simulink library "pfb_library"  (Simulink 6.2)
undefined symbols (not defined in the file or in its folder): add_latency, BitWidthIn, BitWidthOut, bram_latency, buf, CoeffBitWidth, n_inputs, PFBSize, TotalTaps, WindowType
libraries: xbsIndex_r3 x169, pfb_library x11
(part 1 of 2)
settings Model: LastModifiedBy=hchen05

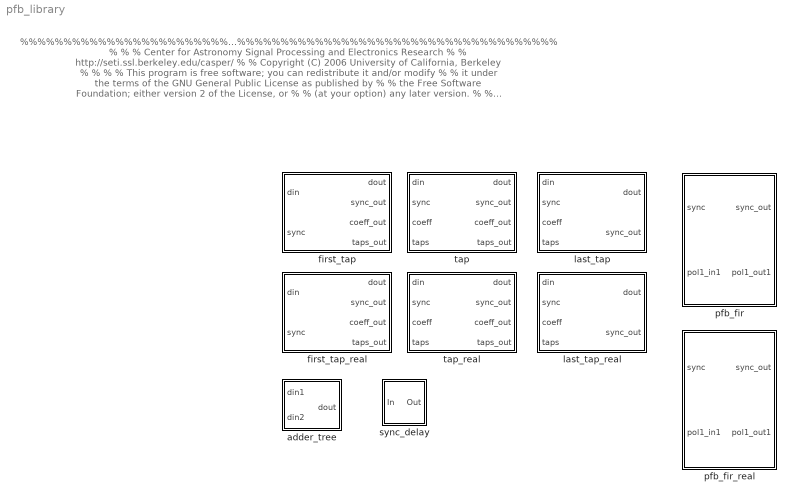
== system pfb_library ==
  note: %%%%%%%%%%%%%%%%%%%%%%%%%%%%%%%%%%%%%%%%%%%%%%%%%%%%%%%%%%%%%%%%%%%%%%%%%%%%%%%
      | %                                                                             %
      | %   Center for Astronomy Signal Processing and Electronics Research           %
      | %   http://seti.ssl.berkeley.edu/casper/                                      %
      | %   Copyright (C) 2006 University of California, Berkeley                     %
      | %                                                                             %
      | %   This program is free software; you can redistribute it and/or modify      %
      | %   it under the terms of the GNU General Public License as published by      %
      | %   the Free Software Foundation; either version 2 of the License, or         %
      | %   (at your option) any later version.                                       %
      | %                                                                             %
      | %   This program is distributed in the hope that it will be useful,           %
      | %   but WITHOUT ANY WARRANTY; without even the implied warranty of            %
      | %   MERCHANTABILITY or FITNESS FOR A PARTICULAR PURPOSE.  See the             %
      | %   GNU General Public License for more details.                              %
      | %                                                                             %
      | %   You should have received a copy of the GNU General Public License along   %
      | %   with this program; if not, write to the Free Software Foundation, Inc.,   %
      | %   51 Franklin Street, Fifth Floor, Boston, MA 02110-1301 USA.               %
      | %                                                                             %
      | %%%%%%%%%%%%%%%%%%%%%%%%%%%%%%%%%%%%%%%%%%%%%%%%%%%%%%%%%%%%%%%%%%%%%%%%%%%%%%%
  adder_tree : Subsystem  mask{num_inputs=2, latency=2}
      mask prompts: num_inputs "Inputs"; latency "Latency per adder tree"
      mask init:
      | adder_tree_mask;
  first_tap : Subsystem  mask(pfb_tap){nput=1, CoeffDistMem=off, fwidth=1}
      mask prompts: nput "This is input number:"; CoeffDistMem "Implement Coefficients in Distributed Memory"; fwidth "Bin Width (normal = 1)"
      mask init:
      | cursys = gcb;
      | disp(cursys);
      | if ~strcmp(get_param([cursys,'/pfb_coeff_gen'], 'CoeffDistMem'), CoeffDistMem),
      |     set_param([cursys,'/pfb_coeff_gen'], 'CoeffDistMem', CoeffDistMem);
      | end
  first_tap_real : Subsystem  mask(pfb_tap_real){nput=1, CoeffDistMem=off, fwidth=1}
      mask prompts: nput "This is input number:"; CoeffDistMem "Implement Coefficients in Distributed Memory"; fwidth "Bin Width (normal = 1)"
      mask init:
      | cursys = gcb;
      | disp(cursys);
      | if ~strcmp(get_param([cursys,'/pfb_coeff_gen'], 'CoeffDistMem'), CoeffDistMem),
      |     set_param([cursys,'/pfb_coeff_gen'], 'CoeffDistMem', CoeffDistMem);
      | end
  last_tap : Subsystem  mask(pfb_tap){quantization=Truncate}
      mask prompts: quantization "Quantization Behavior:"
      mask init:
      | cursys = gcb;
      | disp(cursys);
      | if ~strcmp(get_param([cursys,'/pfb_add_tree'], 'quantization'), quantization),
      |     set_param([cursys,'/pfb_add_tree'], 'quantization', quantization);
      | end
      mask StyleString: popup(Truncate|Round  (unbiased: +/- Inf)|Round  (unbiased: Even Values))
  last_tap_real : Subsystem  mask(pfb_tap_real){quantization=Truncate}
      mask prompts: quantization "Quantization Behavior:"
      mask init:
      | cursys = gcb;
      | disp(cursys);
      | if ~strcmp(get_param([cursys,'/pfb_add_tree'], 'quantization'), quantization),
      |     set_param([cursys,'/pfb_add_tree'], 'quantization', quantization);
      | end
      mask StyleString: popup(Truncate|Round  (unbiased: +/- Inf)|Round  (unbiased: Even Values))
  pfb_fir : Subsystem  mask{PFBSize=5, TotalTaps=2, WindowType=hamming, n_inputs=0, MakeBiplex=off, BitWidthIn=8, BitWidthOut=18, CoeffBitWidth=8, CoeffDistMem=off, add_latency=2, mult_latency=3, bram_latency=2, quantization=Round  (unbiased: +/- Inf), fwidth=1}
      mask prompts: PFBSize "Size of PFB: (2^? pnts)"; TotalTaps "Total Number of Taps:"; WindowType "Windowing Function:"; n_inputs "Number of Simultaneous Inputs: (2^?)"; MakeBiplex "Make Biplex"; BitWidthIn "Input Bitwidth:"; BitWidthOut "Output Bitwidth:"; CoeffBitWidth "Coefficient Bitwidth:"; CoeffDistMem "Use Distributed Memory for Coeffs"; add_latency "Add Latency"; mult_latency "Mult Latency"; bram_latency "BRAM Latency"; quantization "Quantization Behavior"; fwidth "Bin Width Scaling (normal=1)"
      mask init:
      | pfb_fir_mask;
      mask StyleString: edit,edit,popup(bartlett|barthannwin|blackman|blackmanharris|bohamwin|chebwin|flattopwin|gausswin|hamming|hann|kaiser|nuttallwin|parzenwin|rectwin|tukeywin|triang),edit,checkbox,edit,edit,edit,checkbox,edit,edit,edit,popup(Truncate|Round  (unbiased: +/- Inf)|Round  (unbiased: Even Values)),edit
  pfb_fir_real : Subsystem  mask{PFBSize=5, TotalTaps=2, WindowType=hamming, n_inputs=0, MakeBiplex=off, BitWidthIn=8, BitWidthOut=18, CoeffBitWidth=8, CoeffDistMem=off, add_latency=2, mult_latency=3, bram_latency=2, quantization=Round  (unbiased: +/- Inf), fwidth=1}
      mask prompts: PFBSize "Size of PFB: (2^? pnts)"; TotalTaps "Total Number of Taps:"; WindowType "Windowing Function:"; n_inputs "Number of Simultaneous Inputs: (2^?)"; MakeBiplex "Make Biplex"; BitWidthIn "Input Bitwidth:"; BitWidthOut "Output Bitwidth:"; CoeffBitWidth "Coefficient Bitwidth:"; CoeffDistMem "Use Distributed Memory for Coeffs"; add_latency "Add Latency"; mult_latency "Mult Latency"; bram_latency "BRAM Latency"; quantization "Quantization Behavior"; fwidth "Bin Width Scaling (normal=1)"
      mask init:
      | pfb_fir_real_mask;
      mask StyleString: edit,edit,popup(bartlett|barthannwin|blackman|blackmanharris|bohamwin|chebwin|flattopwin|gausswin|hamming|hann|kaiser|nuttallwin|parzenwin|rectwin|tukeywin|triang),edit,checkbox,edit,edit,edit,checkbox,edit,edit,edit,popup(Truncate|Round  (unbiased: +/- Inf)|Round  (unbiased: Even Values)),edit
  sync_delay : Subsystem  mask{DelayLen=4}
      mask prompts: DelayLen "Delay Length:"
      mask init:
      | BitWidth = max(2, ceil(log2(DelayLen+1)));
      | UseCounter = 1;
      | if DelayLen == 0,
      | 	UseCounter = 0;
      | end
      mask Display: fprintf('Z^-%d', DelayLen)
  tap : Subsystem  mask(pfb_tap){}
      mask init:
      | cursys = gcb;
      | disp(cursys);
  tap_real : Subsystem  mask(pfb_tap_real){}
      mask init:
      | cursys = gcb;
      | disp(cursys);

== system pfb_library/adder_tree ==
  din1 : Inport  Port=1  LatchInput=off
  din2 : Inport  Port=2  LatchInput=off
  adder1_1 : xbsIndex_r3/AddSub  mode=Addition  precision=Full  arith_type=Unsigned  n_bits=8  bin_pt=2  quantization=Truncate  overflow=Wrap  latency=latency  explicit_period=on  period=1  use_carryin=off  use_carryout=off  en=off  dbl_ovrd=off  show_param=off  use_core=on  pipeline=on  use_rpm=on  gen_core=off
      settings: xl_area=[0, 0, 0, 0, 0, 0, 0]
  dout : Outport
  wires:
  din1/1 -> adder1_1/1
  din2/1 -> adder1_1/2
  adder1_1/1 -> dout/1

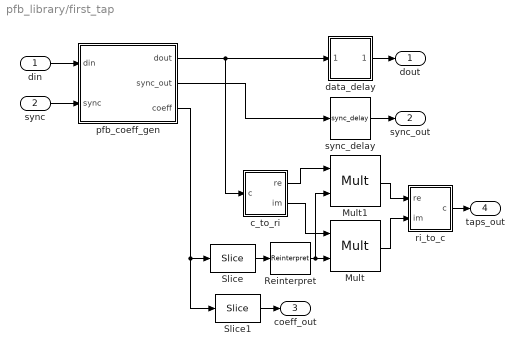
== system pfb_library/first_tap ==
  din : Inport  Port=1  LatchInput=off
  sync : Inport  Port=2  LatchInput=off
  Mult : xbsIndex_r3/Mult  precision=Full  arith_type="Signed  (2's comp)"  n_bits=8  bin_pt=2  quantization=Truncate  overflow=Wrap  latency=mult_latency  explicit_period=off  period=1  en=off  dbl_ovrd=off  show_param=on  mult_type=Parallel  oversample=2  use_embedded=on  pipeline=on  use_rpm=on  placement_style=Rectangular Shape  gen_core=off
      settings: xl_area=[0, 0, 0, 0, 0, 0, 0]
  Mult1 : xbsIndex_r3/Mult  precision=Full  arith_type="Signed  (2's comp)"  n_bits=8  bin_pt=2  quantization=Truncate  overflow=Wrap  latency=mult_latency  explicit_period=off  period=1  en=off  dbl_ovrd=off  show_param=on  mult_type=Parallel  oversample=2  use_embedded=on  pipeline=on  use_rpm=on  placement_style=Rectangular Shape  gen_core=off
      settings: xl_area=[0, 0, 0, 0, 0, 0, 0]
  Reinterpret : xbsIndex_r3/Reinterpret  force_arith_type=on  arith_type="Signed  (2's comp)"  force_bin_pt=on  bin_pt=CoeffBitWidth - 1  force_valid=on
  Slice : xbsIndex_r3/Slice  mode=Lower Bit Location + Width  nbits=CoeffBitWidth  bit1=0  base1=MSB of Input  bit0=0  base0=LSB of Input  boolean_output=off  explicit_period=off  period=1  dbl_ovrd=off
  Slice1 : xbsIndex_r3/Slice  mode=Two Bit Locations  nbits=CoeffBitWidth * (TotalTaps - 1)  bit1=0  base1=MSB of Input  bit0=CoeffBitWidth  base0=LSB of Input  boolean_output=off  explicit_period=off  period=1  dbl_ovrd=off
  c_to_ri : Subsystem
  data_delay : Subsystem
  pfb_coeff_gen : Subsystem  mask{PFBSize=PFBSize, CoeffBitWidth=CoeffBitWidth, TotalTaps=TotalTaps, CoeffDistMem=off, WindowType=WindowType, bram_latency=bram_latency, n_inputs=n_inputs, nput=nput, fwidth=fwidth}
      mask prompts: PFBSize "Size of PFB: (2^? pnts)"; CoeffBitWidth "Bitwidth of Coefficients:"; TotalTaps "Total Number of Taps:"; CoeffDistMem "Implement Coeff Gen in Distributed Memory"; WindowType "Windowing Function:"; bram_latency "BRAM Latency"; n_inputs "Number of Simultaneous Inputs: (2^?)"; nput "This is input number:"; fwidth "Bin Width (normal=1)"
      mask init:
      | pfb_coeff_gen_mask;
  ri_to_c : Subsystem
  sync_delay : pfb_library/sync_delay  DelayLen=2^(PFBSize-n_inputs)
  dout : Outport
  sync_out : Outport  Port=2
  coeff_out : Outport  Port=3
  taps_out : Outport  Port=4
  wires:
  Reinterpret/1 -> Mult/2, Mult1/2
  Slice/1 -> Reinterpret/1
  Slice1/1 -> coeff_out/1
  sync_delay/1 -> sync_out/1
  data_delay/1(Out1) -> dout/1
  din/1 -> pfb_coeff_gen/1(din)
  pfb_coeff_gen/1(dout) -> data_delay/1(In1), c_to_ri/1(c)
  sync/1 -> pfb_coeff_gen/2(sync)
  pfb_coeff_gen/2(sync_out) -> sync_delay/1
  pfb_coeff_gen/3(coeff) -> Slice/1, Slice1/1
  c_to_ri/1(re) -> Mult1/1
  c_to_ri/2(im) -> Mult/1
  Mult1/1 -> ri_to_c/1(re)
  Mult/1 -> ri_to_c/2(im)
  ri_to_c/1(c) -> taps_out/1

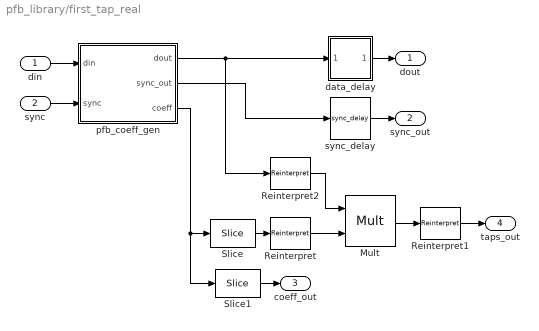
== system pfb_library/first_tap_real ==
  din : Inport  Port=1  LatchInput=off
  sync : Inport  Port=2  LatchInput=off
  Mult : xbsIndex_r3/Mult  precision=Full  arith_type="Signed  (2's comp)"  n_bits=8  bin_pt=2  quantization=Truncate  overflow=Wrap  latency=mult_latency  explicit_period=off  period=1  en=off  dbl_ovrd=off  show_param=on  mult_type=Parallel  oversample=2  use_embedded=on  pipeline=on  use_rpm=on  placement_style=Rectangular Shape  gen_core=off
      settings: xl_area=[0, 0, 0, 0, 0, 0, 0]
  Reinterpret : xbsIndex_r3/Reinterpret  force_arith_type=on  arith_type="Signed  (2's comp)"  force_bin_pt=on  bin_pt=CoeffBitWidth - 1  force_valid=on
  Reinterpret1 : xbsIndex_r3/Reinterpret  force_arith_type=on  arith_type=Unsigned  force_bin_pt=on  bin_pt=0  force_valid=on
  Reinterpret2 : xbsIndex_r3/Reinterpret  force_arith_type=on  arith_type="Signed  (2's comp)"  force_bin_pt=on  bin_pt=BitWidthIn - 1  force_valid=on
  Slice : xbsIndex_r3/Slice  mode=Lower Bit Location + Width  nbits=CoeffBitWidth  bit1=0  base1=MSB of Input  bit0=0  base0=LSB of Input  boolean_output=off  explicit_period=off  period=1  dbl_ovrd=off
  Slice1 : xbsIndex_r3/Slice  mode=Two Bit Locations  nbits=CoeffBitWidth * (TotalTaps - 1)  bit1=0  base1=MSB of Input  bit0=CoeffBitWidth  base0=LSB of Input  boolean_output=off  explicit_period=off  period=1  dbl_ovrd=off
  data_delay : Subsystem
  pfb_coeff_gen : Subsystem  mask{PFBSize=PFBSize, CoeffBitWidth=CoeffBitWidth, TotalTaps=TotalTaps, CoeffDistMem=off, WindowType=WindowType, bram_latency=bram_latency, n_inputs=n_inputs, nput=nput, fwidth=fwidth}
      mask prompts: PFBSize "Size of PFB: (2^? pnts)"; CoeffBitWidth "Bitwidth of Coefficients:"; TotalTaps "Total Number of Taps:"; CoeffDistMem "Implement Coeff Gen in Distributed Memory"; WindowType "Windowing Function:"; bram_latency "BRAM Latency"; n_inputs "Number of Simultaneous Inputs: (2^?)"; nput "This is input number:"; fwidth "Bin Width (normal=1)"
      mask init:
      | pfb_coeff_gen_mask;
  sync_delay : pfb_library/sync_delay  DelayLen=2^(PFBSize-n_inputs)
  dout : Outport
  sync_out : Outport  Port=2
  coeff_out : Outport  Port=3
  taps_out : Outport  Port=4
  wires:
  Mult/1 -> Reinterpret1/1
  pfb_coeff_gen/3(coeff) -> Slice1/1, Slice/1
  pfb_coeff_gen/2(sync_out) -> sync_delay/1
  sync/1 -> pfb_coeff_gen/2(sync)
  pfb_coeff_gen/1(dout) -> data_delay/1(In1), Reinterpret2/1
  din/1 -> pfb_coeff_gen/1(din)
  data_delay/1(Out1) -> dout/1
  sync_delay/1 -> sync_out/1
  Slice1/1 -> coeff_out/1
  Slice/1 -> Reinterpret/1
  Reinterpret/1 -> Mult/2
  Reinterpret1/1 -> taps_out/1
  Reinterpret2/1 -> Mult/1

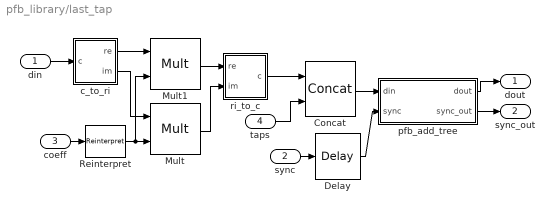
== system pfb_library/last_tap ==
  din : Inport  Port=1  LatchInput=off
  sync : Inport  Port=2  LatchInput=off
  coeff : Inport  Port=3  LatchInput=off
  taps : Inport  Port=4  LatchInput=off
  Concat : xbsIndex_r3/Concat  num_inputs=2  explicit_period=off  period=1  dbl_ovrd=off
  Delay : xbsIndex_r3/Delay  latency=mult_latency  reg_retiming=off  explicit_period=off  period=1  en=off  accept_only_valid=off  init_zero=on  dbl_ovrd=off  show_param=off
      settings: xl_area=[0, 0, 0, 0, 0, 0, 0]
  Mult : xbsIndex_r3/Mult  precision=Full  arith_type="Signed  (2's comp)"  n_bits=8  bin_pt=2  quantization=Truncate  overflow=Wrap  latency=mult_latency  explicit_period=off  period=1  en=off  dbl_ovrd=off  show_param=on  mult_type=Parallel  oversample=2  use_embedded=on  pipeline=on  use_rpm=on  placement_style=Rectangular Shape  gen_core=off
      settings: xl_area=[0, 0, 0, 0, 0, 0, 0]
  Mult1 : xbsIndex_r3/Mult  precision=Full  arith_type="Signed  (2's comp)"  n_bits=8  bin_pt=2  quantization=Truncate  overflow=Wrap  latency=mult_latency  explicit_period=off  period=1  en=off  dbl_ovrd=off  show_param=on  mult_type=Parallel  oversample=2  use_embedded=on  pipeline=on  use_rpm=on  placement_style=Rectangular Shape  gen_core=off
      settings: xl_area=[0, 0, 0, 0, 0, 0, 0]
  Reinterpret : xbsIndex_r3/Reinterpret  force_arith_type=on  arith_type="Signed  (2's comp)"  force_bin_pt=on  bin_pt=CoeffBitWidth - 1  force_valid=on
  c_to_ri : Subsystem
  pfb_add_tree : Subsystem  mask{TotalTaps=TotalTaps, BitWidthIn=BitWidthIn, BitWidthOut=BitWidthOut, CoeffBitWidth=CoeffBitWidth, add_latency=add_latency, quantization=Truncate}
      mask prompts: TotalTaps "Total Number of Taps:"; BitWidthIn "Input Bitwidth:"; BitWidthOut "Output Bitwidth:"; CoeffBitWidth "Coeff Bitwidth:"; add_latency "Add Latency"; quantization "Quantization Behavior"
      mask init:
      | pfb_add_mask;
      mask StyleString: edit,edit,edit,edit,edit,popup(Truncate|Round  (unbiased: +/- Inf)|Round  (unbiased: Even Values))
  ri_to_c : Subsystem
  dout : Outport
  sync_out : Outport  Port=2
  wires:
  Reinterpret/1 -> Mult/2, Mult1/2
  coeff/1 -> Reinterpret/1
  Concat/1 -> pfb_add_tree/1(din)
  taps/1 -> Concat/2
  sync/1 -> Delay/1
  pfb_add_tree/1(dout) -> dout/1
  pfb_add_tree/2(sync_out) -> sync_out/1
  Delay/1 -> pfb_add_tree/2(sync)
  c_to_ri/1(re) -> Mult1/1
  c_to_ri/2(im) -> Mult/1
  din/1 -> c_to_ri/1(c)
  Mult1/1 -> ri_to_c/1(re)
  Mult/1 -> ri_to_c/2(im)
  ri_to_c/1(c) -> Concat/1

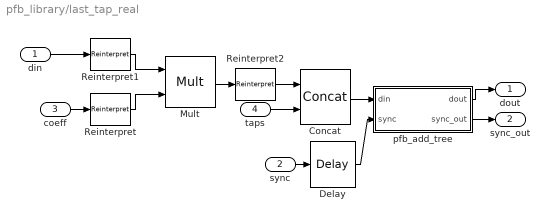
== system pfb_library/last_tap_real ==
  din : Inport  Port=1  LatchInput=off
  sync : Inport  Port=2  LatchInput=off
  coeff : Inport  Port=3  LatchInput=off
  taps : Inport  Port=4  LatchInput=off
  Concat : xbsIndex_r3/Concat  num_inputs=2  explicit_period=off  period=1  dbl_ovrd=off
  Delay : xbsIndex_r3/Delay  latency=mult_latency  reg_retiming=off  explicit_period=off  period=1  en=off  accept_only_valid=off  init_zero=on  dbl_ovrd=off  show_param=off
      settings: xl_area=[0, 0, 0, 0, 0, 0, 0]
  Mult : xbsIndex_r3/Mult  precision=Full  arith_type="Signed  (2's comp)"  n_bits=8  bin_pt=2  quantization=Truncate  overflow=Wrap  latency=mult_latency  explicit_period=off  period=1  en=off  dbl_ovrd=off  show_param=on  mult_type=Parallel  oversample=2  use_embedded=on  pipeline=on  use_rpm=on  placement_style=Rectangular Shape  gen_core=off
      settings: xl_area=[0, 0, 0, 0, 0, 0, 0]
  Reinterpret : xbsIndex_r3/Reinterpret  force_arith_type=on  arith_type="Signed  (2's comp)"  force_bin_pt=on  bin_pt=CoeffBitWidth - 1  force_valid=on
  Reinterpret1 : xbsIndex_r3/Reinterpret  force_arith_type=on  arith_type="Signed  (2's comp)"  force_bin_pt=on  bin_pt=BitWidthIn - 1  force_valid=on
  Reinterpret2 : xbsIndex_r3/Reinterpret  force_arith_type=on  arith_type=Unsigned  force_bin_pt=on  bin_pt=0  force_valid=on
  pfb_add_tree : Subsystem  mask{TotalTaps=TotalTaps, BitWidthIn=BitWidthIn, BitWidthOut=BitWidthOut, CoeffBitWidth=CoeffBitWidth, add_latency=add_latency, quantization=Truncate}
      mask prompts: TotalTaps "Total Number of Taps:"; BitWidthIn "Input Bitwidth:"; BitWidthOut "Output Bitwidth:"; CoeffBitWidth "Coeff Bitwidth:"; add_latency "Add Latency"; quantization "Quantization Behavior"
      mask init:
      | pfb_add_real_mask;
      mask StyleString: edit,edit,edit,edit,edit,popup(Truncate|Round  (unbiased: +/- Inf)|Round  (unbiased: Even Values))
  dout : Outport
  sync_out : Outport  Port=2
  wires:
  din/1 -> Reinterpret1/1
  Delay/1 -> pfb_add_tree/2(sync)
  pfb_add_tree/2(sync_out) -> sync_out/1
  pfb_add_tree/1(dout) -> dout/1
  sync/1 -> Delay/1
  taps/1 -> Concat/2
  Concat/1 -> pfb_add_tree/1(din)
  coeff/1 -> Reinterpret/1
  Reinterpret/1 -> Mult/2
  Mult/1 -> Reinterpret2/1
  Reinterpret1/1 -> Mult/1
  Reinterpret2/1 -> Concat/1

== system pfb_library/pfb_fir ==
  sync : Inport  Port=1  LatchInput=off
  pol1_in1 : Inport  Port=2  LatchInput=off
  pol1_in1_first_tap : pfb_library/first_tap  nput=0  CoeffDistMem=off  fwidth=1
  pol1_in1_last_tap : pfb_library/last_tap  quantization="Round  (unbiased: +/- Inf)"
  sync_out : Outport
  pol1_out1 : Outport  Port=2
  wires:
  pol1_in1/1 -> pol1_in1_first_tap/1
  sync/1 -> pol1_in1_first_tap/2
  pol1_in1_first_tap/1 -> pol1_in1_last_tap/1
  pol1_in1_first_tap/2 -> pol1_in1_last_tap/2
  pol1_in1_first_tap/3 -> pol1_in1_last_tap/3
  pol1_in1_first_tap/4 -> pol1_in1_last_tap/4
  pol1_in1_last_tap/1 -> pol1_out1/1
  pol1_in1_last_tap/2 -> sync_out/1

== system pfb_library/pfb_fir_real ==
  sync : Inport  Port=1  LatchInput=off
  pol1_in1 : Inport  Port=2  LatchInput=off
  pol1_in1_first_tap : pfb_library/first_tap_real  nput=0  CoeffDistMem=off  fwidth=fwidth
  pol1_in1_last_tap : pfb_library/last_tap_real  quantization="Round  (unbiased: +/- Inf)"
  sync_out : Outport
  pol1_out1 : Outport  Port=2
  wires:
  pol1_in1/1 -> pol1_in1_first_tap/1
  sync/1 -> pol1_in1_first_tap/2
  pol1_in1_first_tap/1 -> pol1_in1_last_tap/1
  pol1_in1_first_tap/2 -> pol1_in1_last_tap/2
  pol1_in1_first_tap/3 -> pol1_in1_last_tap/3
  pol1_in1_first_tap/4 -> pol1_in1_last_tap/4
  pol1_in1_last_tap/1 -> pol1_out1/1
  pol1_in1_last_tap/2 -> sync_out/1

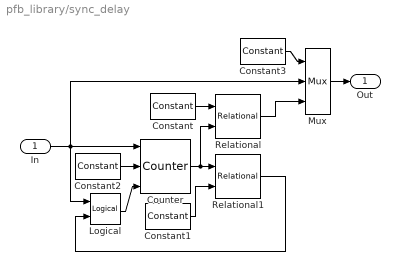
== system pfb_library/sync_delay ==
  In : Inport  Port=1  LatchInput=off
  Constant : xbsIndex_r3/Constant  const=1  equ=P=C  arith_type=Unsigned  n_bits=BitWidth  bin_pt=0  opselect=C  inp2=PCIN>>17  opr=+  inp1=P  carry=CIN  iostate=0  explicit_period=on  period=1  dbl_ovrd=off
  Constant1 : xbsIndex_r3/Constant  const=0  equ=P=C  arith_type=Unsigned  n_bits=BitWidth  bin_pt=0  opselect=C  inp2=PCIN>>17  opr=+  inp1=P  carry=CIN  iostate=0  explicit_period=on  period=1  dbl_ovrd=off
  Constant2 : xbsIndex_r3/Constant  const=DelayLen  equ=P=C  arith_type=Unsigned  n_bits=BitWidth  bin_pt=0  opselect=C  inp2=PCIN>>17  opr=+  inp1=P  carry=CIN  iostate=0  explicit_period=on  period=1  dbl_ovrd=off
  Constant3 : xbsIndex_r3/Constant  const=UseCounter  equ=P=C  arith_type=Unsigned  n_bits=1  bin_pt=0  opselect=C  inp2=PCIN>>17  opr=+  inp1=P  carry=CIN  iostate=0  explicit_period=on  period=1  dbl_ovrd=off
  Counter : xbsIndex_r3/Counter  cnt_type=Free Running  n_bits=BitWidth  bin_pt=0  arith_type=Unsigned  start_count=0  cnt_to=Inf  cnt_by_val=1  operation=Down  explicit_period=on  period=1  load_pin=on  rst=off  en=on  dbl_ovrd=off  show_param=off  use_rpm=on  gen_core=off
      settings: xl_area=[0, 0, 0, 0, 0, 0, 0]
  Logical : xbsIndex_r3/Logical  logical_function=OR  inputs=2  precision=Full  arith_type=Unsigned  n_bits=8  bin_pt=2  align_bp=on  latency=0  explicit_period=on  period=1  en=off  dbl_ovrd=off  show_param=off
      settings: xl_area=[0, 0, 0, 0, 0, 0, 0]
  Mux : xbsIndex_r3/Mux  inputs=2  precision=Full  arith_type="Signed  (2's comp)"  n_bits=8  bin_pt=2  quantization=Truncate  overflow=Wrap  latency=0  explicit_period=off  period=1  en=off  dbl_ovrd=off  show_param=off  mux_type=off  use_rpm=off  gen_core=off
      settings: xl_area=[0, 0, 0, 0, 0, 0, 0]
  Relational : xbsIndex_r3/Relational  mode=a=b  latency=0  explicit_period=off  period=1  en=off  dbl_ovrd=off  show_param=off
      settings: xl_area=[0, 0, 0, 0, 0, 0, 0]
  Relational1 : xbsIndex_r3/Relational  mode=a!=b  latency=0  explicit_period=on  period=1  en=off  dbl_ovrd=off  show_param=off
      settings: xl_area=[0, 0, 0, 0, 0, 0, 0]
  Out : Outport
  wires:
  Counter/1 -> Relational1/1, Relational/2
  Constant1/1 -> Relational1/2
  Constant/1 -> Relational/1
  Constant2/1 -> Counter/2
  In/1 -> Counter/1, Logical/1, Mux/2
  Logical/1 -> Counter/3
  Relational1/1 -> Logical/2
  Relational/1 -> Mux/3
  Constant3/1 -> Mux/1
  Mux/1 -> Out/1

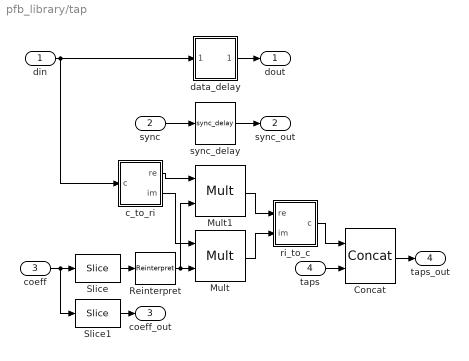
== system pfb_library/tap ==
  din : Inport  Port=1  LatchInput=off
  sync : Inport  Port=2  LatchInput=off
  coeff : Inport  Port=3  LatchInput=off
  taps : Inport  Port=4  LatchInput=off
  Concat : xbsIndex_r3/Concat  num_inputs=2  explicit_period=off  period=1  dbl_ovrd=off
  Mult : xbsIndex_r3/Mult  precision=Full  arith_type="Signed  (2's comp)"  n_bits=8  bin_pt=2  quantization=Truncate  overflow=Wrap  latency=mult_latency  explicit_period=off  period=1  en=off  dbl_ovrd=off  show_param=on  mult_type=Parallel  oversample=2  use_embedded=on  pipeline=on  use_rpm=on  placement_style=Rectangular Shape  gen_core=off
      settings: xl_area=[0, 0, 0, 0, 0, 0, 0]
  Mult1 : xbsIndex_r3/Mult  precision=Full  arith_type="Signed  (2's comp)"  n_bits=8  bin_pt=2  quantization=Truncate  overflow=Wrap  latency=mult_latency  explicit_period=off  period=1  en=off  dbl_ovrd=off  show_param=on  mult_type=Parallel  oversample=2  use_embedded=on  pipeline=on  use_rpm=on  placement_style=Rectangular Shape  gen_core=off
      settings: xl_area=[0, 0, 0, 0, 0, 0, 0]
  Reinterpret : xbsIndex_r3/Reinterpret  force_arith_type=on  arith_type="Signed  (2's comp)"  force_bin_pt=on  bin_pt=CoeffBitWidth - 1  force_valid=on
  Slice : xbsIndex_r3/Slice  mode=Lower Bit Location + Width  nbits=CoeffBitWidth  bit1=0  base1=MSB of Input  bit0=0  base0=LSB of Input  boolean_output=off  explicit_period=off  period=1  dbl_ovrd=off
  Slice1 : xbsIndex_r3/Slice  mode=Two Bit Locations  nbits=0  bit1=0  base1=MSB of Input  bit0=CoeffBitWidth  base0=LSB of Input  boolean_output=off  explicit_period=off  period=1  dbl_ovrd=off
  c_to_ri : Subsystem
  data_delay : Subsystem
  ri_to_c : Subsystem
  sync_delay : pfb_library/sync_delay  DelayLen=2^(PFBSize-n_inputs)
  dout : Outport
  sync_out : Outport  Port=2
  coeff_out : Outport  Port=3
  taps_out : Outport  Port=4
  wires:
  Reinterpret/1 -> Mult/2, Mult1/2
  Slice/1 -> Reinterpret/1
  Slice1/1 -> coeff_out/1
  coeff/1 -> Slice1/1, Slice/1
  Concat/1 -> taps_out/1
  taps/1 -> Concat/2
  sync_delay/1 -> sync_out/1
  sync/1 -> sync_delay/1
  Mult1/1 -> ri_to_c/1(re)
  Mult/1 -> ri_to_c/2(im)
  ri_to_c/1(c) -> Concat/1
  c_to_ri/1(re) -> Mult1/1
  c_to_ri/2(im) -> Mult/1
  din/1 -> data_delay/1(In1), c_to_ri/1(c)
  data_delay/1(Out1) -> dout/1

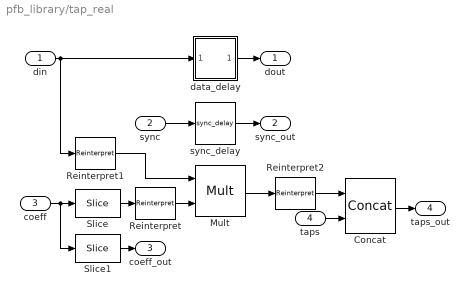
== system pfb_library/tap_real ==
  din : Inport  Port=1  LatchInput=off
  sync : Inport  Port=2  LatchInput=off
  coeff : Inport  Port=3  LatchInput=off
  taps : Inport  Port=4  LatchInput=off
  Concat : xbsIndex_r3/Concat  num_inputs=2  explicit_period=off  period=1  dbl_ovrd=off
  Mult : xbsIndex_r3/Mult  precision=Full  arith_type="Signed  (2's comp)"  n_bits=8  bin_pt=2  quantization=Truncate  overflow=Wrap  latency=mult_latency  explicit_period=off  period=1  en=off  dbl_ovrd=off  show_param=on  mult_type=Parallel  oversample=2  use_embedded=on  pipeline=on  use_rpm=on  placement_style=Rectangular Shape  gen_core=off
      settings: xl_area=[0, 0, 0, 0, 0, 0, 0]
  Reinterpret : xbsIndex_r3/Reinterpret  force_arith_type=on  arith_type="Signed  (2's comp)"  force_bin_pt=on  bin_pt=CoeffBitWidth - 1  force_valid=on
  Reinterpret1 : xbsIndex_r3/Reinterpret  force_arith_type=on  arith_type="Signed  (2's comp)"  force_bin_pt=on  bin_pt=BitWidthIn - 1  force_valid=on
  Reinterpret2 : xbsIndex_r3/Reinterpret  force_arith_type=on  arith_type=Unsigned  force_bin_pt=on  bin_pt=0  force_valid=on
  Slice : xbsIndex_r3/Slice  mode=Lower Bit Location + Width  nbits=CoeffBitWidth  bit1=0  base1=MSB of Input  bit0=0  base0=LSB of Input  boolean_output=off  explicit_period=off  period=1  dbl_ovrd=off
  Slice1 : xbsIndex_r3/Slice  mode=Two Bit Locations  nbits=0  bit1=0  base1=MSB of Input  bit0=CoeffBitWidth  base0=LSB of Input  boolean_output=off  explicit_period=off  period=1  dbl_ovrd=off
  data_delay : Subsystem
  sync_delay : pfb_library/sync_delay  DelayLen=2^(PFBSize-n_inputs)
  dout : Outport
  sync_out : Outport  Port=2
  coeff_out : Outport  Port=3
  taps_out : Outport  Port=4
  wires:
  data_delay/1(Out1) -> dout/1
  din/1 -> data_delay/1(In1), Reinterpret1/1
  Mult/1 -> Reinterpret2/1
  sync/1 -> sync_delay/1
  sync_delay/1 -> sync_out/1
  taps/1 -> Concat/2
  Concat/1 -> taps_out/1
  coeff/1 -> Slice/1, Slice1/1
  Slice1/1 -> coeff_out/1
  Slice/1 -> Reinterpret/1
  Reinterpret/1 -> Mult/2
  Reinterpret1/1 -> Mult/1
  Reinterpret2/1 -> Concat/1

== system pfb_library/first_tap/c_to_ri ==
  c : Inport  Port=1  LatchInput=off
  Reinterpret : xbsIndex_r3/Reinterpret  force_arith_type=on  arith_type="Signed  (2's comp)"  force_bin_pt=on  bin_pt=BitWidthIn - 1  force_valid=on
  Reinterpret1 : xbsIndex_r3/Reinterpret  force_arith_type=on  arith_type="Signed  (2's comp)"  force_bin_pt=on  bin_pt=BitWidthIn - 1  force_valid=on
  Slice : xbsIndex_r3/Slice  mode=Upper Bit Location + Width  nbits=BitWidthIn  bit1=0  base1=MSB of Input  bit0=0  base0=LSB of Input  boolean_output=off  explicit_period=off  period=1  dbl_ovrd=off
  Slice1 : xbsIndex_r3/Slice  mode=Lower Bit Location + Width  nbits=BitWidthIn  bit1=0  base1=MSB of Input  bit0=0  base0=LSB of Input  boolean_output=off  explicit_period=off  period=1  dbl_ovrd=off
  re : Outport
  im : Outport  Port=2
  wires:
  c/1 -> Slice1/1, Slice/1
  Reinterpret1/1 -> im/1
  Reinterpret/1 -> re/1
  Slice1/1 -> Reinterpret1/1
  Slice/1 -> Reinterpret/1

== system pfb_library/first_tap/data_delay ==
  In1 : Inport  Port=1  LatchInput=off
  Constant2 : xbsIndex_r3/Constant  const=1  equ=P=C  arith_type=Boolean  n_bits=1  bin_pt=0  opselect=C  inp2=PCIN>>17  opr=+  inp1=P  carry=CIN  iostate=0  explicit_period=on  period=1  dbl_ovrd=off
  Counter : xbsIndex_r3/Counter  cnt_type=Count Limited  n_bits=PFBSize-n_inputs  bin_pt=0  arith_type=Unsigned  start_count=0  cnt_to=2^(PFBSize-n_inputs) - bram_latency - 1  cnt_by_val=1  operation=Up  explicit_period=off  period=1  load_pin=off  rst=off  en=off  dbl_ovrd=off  show_param=off  use_rpm=off  gen_core=on
      settings: xl_area=[0, 0, 0, 0, 0, 0, 0]
  Single Port RAM : xbsIndex_r3/Single Port RAM  depth=2^(PFBSize-n_inputs)  initVector=0  write_mode=Read Before Write  latency=bram_latency  init_zero=on  explicit_period=off  period=1  rst=off  init_reg=0  en=off  dbl_ovrd=off  show_param=off  distributed_mem=off  use_rpm=off  gen_core=off
      settings: xl_area=[0, 0, 0, 0, 0, 0, 0]
  Out1 : Outport
  wires:
  Single Port RAM/1 -> Out1/1
  Counter/1 -> Single Port RAM/1
  In1/1 -> Single Port RAM/2
  Constant2/1 -> Single Port RAM/3

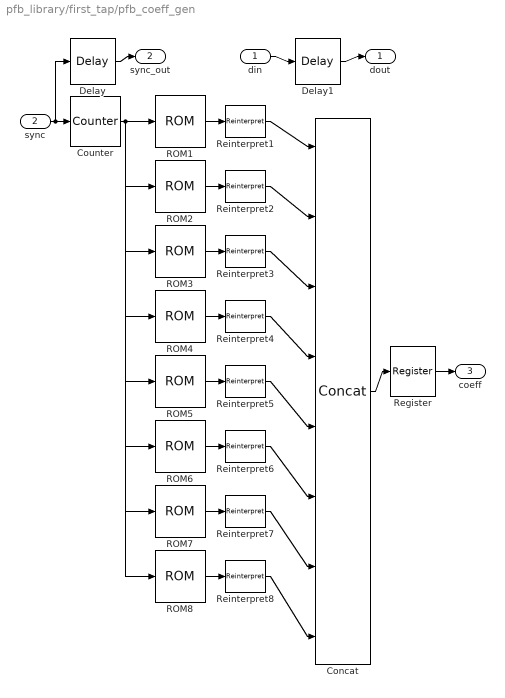
== system pfb_library/first_tap/pfb_coeff_gen ==
  din : Inport  Port=1  LatchInput=off
  sync : Inport  Port=2  LatchInput=off
  Concat : xbsIndex_r3/Concat  num_inputs=8  explicit_period=off  period=1  dbl_ovrd=off
  Counter : xbsIndex_r3/Counter  cnt_type=Free Running  n_bits=PFBSize-n_inputs  bin_pt=0  arith_type=Unsigned  start_count=0  cnt_to=Inf  cnt_by_val=1  operation=Up  explicit_period=on  period=1  load_pin=off  rst=on  en=off  dbl_ovrd=off  show_param=off  use_rpm=on  gen_core=off
      settings: xl_area=[0, 0, 0, 0, 0, 0, 0]
  Delay : xbsIndex_r3/Delay  latency=bram_latency+1  reg_retiming=off  explicit_period=off  period=1  en=off  accept_only_valid=off  init_zero=on  dbl_ovrd=off  show_param=off
      settings: xl_area=[0, 0, 0, 0, 0, 0, 0]
  Delay1 : xbsIndex_r3/Delay  latency=bram_latency+1  reg_retiming=off  explicit_period=off  period=1  en=off  accept_only_valid=off  init_zero=on  dbl_ovrd=off  show_param=off
      settings: xl_area=[0, 0, 0, 0, 0, 0, 0]
  ROM1 : xbsIndex_r3/ROM  depth=2^(PFBSize-n_inputs)  initVector=buf(0*2^(PFBSize-n_inputs) + 1:1*2^(PFBSize-n_inputs))  arith_type="Signed  (2's comp)"  n_bits=CoeffBitWidth  bin_pt=CoeffBitWidth-1  latency=bram_latency  init_zero=on  explicit_period=off  period=1  rst=off  init_reg=0  en=off  dbl_ovrd=off  show_param=on  distributed_mem=on  use_rpm=off  gen_core=off
      settings: xl_area=[0, 0, 0, 0, 0, 0, 0]
  ROM2 : xbsIndex_r3/ROM  depth=2^(PFBSize-n_inputs)  initVector=buf(1*2^(PFBSize-n_inputs) + 1:2*2^(PFBSize-n_inputs))  arith_type="Signed  (2's comp)"  n_bits=CoeffBitWidth  bin_pt=CoeffBitWidth-1  latency=bram_latency  init_zero=on  explicit_period=off  period=1  rst=off  init_reg=0  en=off  dbl_ovrd=off  show_param=on  distributed_mem=on  use_rpm=off  gen_core=off
      settings: xl_area=[0, 0, 0, 0, 0, 0, 0]
  ROM3 : xbsIndex_r3/ROM  depth=2^(PFBSize-n_inputs)  initVector=buf(2*2^(PFBSize-n_inputs) + 1:3*2^(PFBSize-n_inputs))  arith_type="Signed  (2's comp)"  n_bits=CoeffBitWidth  bin_pt=CoeffBitWidth-1  latency=bram_latency  init_zero=on  explicit_period=off  period=1  rst=off  init_reg=0  en=off  dbl_ovrd=off  show_param=on  distributed_mem=on  use_rpm=off  gen_core=off
      settings: xl_area=[0, 0, 0, 0, 0, 0, 0]
  ROM4 : xbsIndex_r3/ROM  depth=2^(PFBSize-n_inputs)  initVector=buf(3*2^(PFBSize-n_inputs) + 1:4*2^(PFBSize-n_inputs))  arith_type="Signed  (2's comp)"  n_bits=CoeffBitWidth  bin_pt=CoeffBitWidth-1  latency=bram_latency  init_zero=on  explicit_period=off  period=1  rst=off  init_reg=0  en=off  dbl_ovrd=off  show_param=on  distributed_mem=on  use_rpm=off  gen_core=off
      settings: xl_area=[0, 0, 0, 0, 0, 0, 0]
  ROM5 : xbsIndex_r3/ROM  depth=2^(PFBSize-n_inputs)  initVector=buf(4*2^(PFBSize-n_inputs) + 1:5*2^(PFBSize-n_inputs))  arith_type="Signed  (2's comp)"  n_bits=CoeffBitWidth  bin_pt=CoeffBitWidth-1  latency=bram_latency  init_zero=on  explicit_period=off  period=1  rst=off  init_reg=0  en=off  dbl_ovrd=off  show_param=on  distributed_mem=on  use_rpm=off  gen_core=off
      settings: xl_area=[0, 0, 0, 0, 0, 0, 0]
  ROM6 : xbsIndex_r3/ROM  depth=2^(PFBSize-n_inputs)  initVector=buf(5*2^(PFBSize-n_inputs) + 1:6*2^(PFBSize-n_inputs))  arith_type="Signed  (2's comp)"  n_bits=CoeffBitWidth  bin_pt=CoeffBitWidth-1  latency=bram_latency  init_zero=on  explicit_period=off  period=1  rst=off  init_reg=0  en=off  dbl_ovrd=off  show_param=on  distributed_mem=on  use_rpm=off  gen_core=off
      settings: xl_area=[0, 0, 0, 0, 0, 0, 0]
  ROM7 : xbsIndex_r3/ROM  depth=2^(PFBSize-n_inputs)  initVector=buf(6*2^(PFBSize-n_inputs) + 1:7*2^(PFBSize-n_inputs))  arith_type="Signed  (2's comp)"  n_bits=CoeffBitWidth  bin_pt=CoeffBitWidth-1  latency=bram_latency  init_zero=on  explicit_period=off  period=1  rst=off  init_reg=0  en=off  dbl_ovrd=off  show_param=on  distributed_mem=on  use_rpm=off  gen_core=off
      settings: xl_area=[0, 0, 0, 0, 0, 0, 0]
  ROM8 : xbsIndex_r3/ROM  depth=2^(PFBSize-n_inputs)  initVector=buf(7*2^(PFBSize-n_inputs) + 1:8*2^(PFBSize-n_inputs))  arith_type="Signed  (2's comp)"  n_bits=CoeffBitWidth  bin_pt=CoeffBitWidth-1  latency=bram_latency  init_zero=on  explicit_period=off  period=1  rst=off  init_reg=0  en=off  dbl_ovrd=off  show_param=on  distributed_mem=on  use_rpm=off  gen_core=off
      settings: xl_area=[0, 0, 0, 0, 0, 0, 0]
  Register : xbsIndex_r3/Register  init=0  reg_only_valid=off  explicit_period=off  period=1  rst=off  en=off  out_en=off  dbl_ovrd=off  show_param=off
      settings: xl_area=[0, 0, 0, 0, 0, 0, 0]
  Reinterpret{1..8} (8 alike) : xbsIndex_r3/Reinterpret  force_arith_type=on  arith_type=Unsigned  force_bin_pt=on  bin_pt=0  force_valid=on
  dout : Outport
  sync_out : Outport  Port=2
  coeff : Outport  Port=3
  wires:
  din/1 -> Delay1/1
  Delay1/1 -> dout/1
  sync/1 -> Counter/1, Delay/1
  Delay/1 -> sync_out/1
  Concat/1 -> Register/1
  Register/1 -> coeff/1
  Counter/1 -> ROM1/1, ROM2/1, ROM3/1, ROM4/1, ROM5/1, ROM6/1, ROM7/1, ROM8/1
  ROM1/1 -> Reinterpret1/1
  Reinterpret1/1 -> Concat/1
  ROM2/1 -> Reinterpret2/1
  Reinterpret2/1 -> Concat/2
  ROM3/1 -> Reinterpret3/1
  Reinterpret3/1 -> Concat/3
  ROM4/1 -> Reinterpret4/1
  Reinterpret4/1 -> Concat/4
  ROM5/1 -> Reinterpret5/1
  Reinterpret5/1 -> Concat/5
  ROM6/1 -> Reinterpret6/1
  Reinterpret6/1 -> Concat/6
  ROM7/1 -> Reinterpret7/1
  Reinterpret7/1 -> Concat/7
  ROM8/1 -> Reinterpret8/1
  Reinterpret8/1 -> Concat/8

== system pfb_library/first_tap/ri_to_c ==
  re : Inport  Port=1  LatchInput=off
  im : Inport  Port=2  LatchInput=off
  Concat : xbsIndex_r3/Concat  num_inputs=2  explicit_period=off  period=1  dbl_ovrd=off
  Reinterpret : xbsIndex_r3/Reinterpret  force_arith_type=on  arith_type=Unsigned  force_bin_pt=on  bin_pt=0  force_valid=on
  Reinterpret1 : xbsIndex_r3/Reinterpret  force_arith_type=on  arith_type=Unsigned  force_bin_pt=on  bin_pt=0  force_valid=on
  c : Outport
  wires:
  im/1 -> Reinterpret1/1
  Concat/1 -> c/1
  re/1 -> Reinterpret/1
  Reinterpret1/1 -> Concat/2
  Reinterpret/1 -> Concat/1

== system pfb_library/first_tap_real/data_delay ==
  In1 : Inport  Port=1  LatchInput=off
  Constant2 : xbsIndex_r3/Constant  const=1  equ=P=C  arith_type=Boolean  n_bits=1  bin_pt=0  opselect=C  inp2=PCIN>>17  opr=+  inp1=P  carry=CIN  iostate=0  explicit_period=on  period=1  dbl_ovrd=off
  Counter : xbsIndex_r3/Counter  cnt_type=Count Limited  n_bits=PFBSize-n_inputs  bin_pt=0  arith_type=Unsigned  start_count=0  cnt_to=2^(PFBSize-n_inputs) - bram_latency - 1  cnt_by_val=1  operation=Up  explicit_period=off  period=1  load_pin=off  rst=off  en=off  dbl_ovrd=off  show_param=off  use_rpm=off  gen_core=on
      settings: xl_area=[0, 0, 0, 0, 0, 0, 0]
  Single Port RAM : xbsIndex_r3/Single Port RAM  depth=2^(PFBSize-n_inputs)  initVector=0  write_mode=Read Before Write  latency=bram_latency  init_zero=on  explicit_period=off  period=1  rst=off  init_reg=0  en=off  dbl_ovrd=off  show_param=off  distributed_mem=off  use_rpm=off  gen_core=off
      settings: xl_area=[0, 0, 0, 0, 0, 0, 0]
  Out1 : Outport
  wires:
  Constant2/1 -> Single Port RAM/3
  In1/1 -> Single Port RAM/2
  Counter/1 -> Single Port RAM/1
  Single Port RAM/1 -> Out1/1

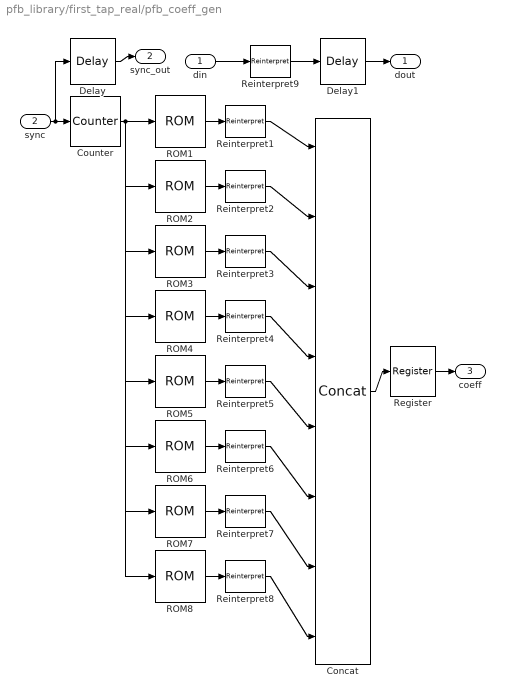
== system pfb_library/first_tap_real/pfb_coeff_gen ==
  din : Inport  Port=1  LatchInput=off
  sync : Inport  Port=2  LatchInput=off
  Concat : xbsIndex_r3/Concat  num_inputs=8  explicit_period=off  period=1  dbl_ovrd=off
  Counter : xbsIndex_r3/Counter  cnt_type=Free Running  n_bits=PFBSize-n_inputs  bin_pt=0  arith_type=Unsigned  start_count=0  cnt_to=Inf  cnt_by_val=1  operation=Up  explicit_period=on  period=1  load_pin=off  rst=on  en=off  dbl_ovrd=off  show_param=off  use_rpm=on  gen_core=off
      settings: xl_area=[0, 0, 0, 0, 0, 0, 0]
  Delay : xbsIndex_r3/Delay  latency=bram_latency+1  reg_retiming=off  explicit_period=off  period=1  en=off  accept_only_valid=off  init_zero=on  dbl_ovrd=off  show_param=off
      settings: xl_area=[0, 0, 0, 0, 0, 0, 0]
  Delay1 : xbsIndex_r3/Delay  latency=bram_latency+1  reg_retiming=off  explicit_period=off  period=1  en=off  accept_only_valid=off  init_zero=on  dbl_ovrd=off  show_param=off
      settings: xl_area=[0, 0, 0, 0, 0, 0, 0]
  ROM1 : xbsIndex_r3/ROM  depth=2^(PFBSize-n_inputs)  initVector=buf(0*2^(PFBSize-n_inputs) + 1:1*2^(PFBSize-n_inputs))  arith_type="Signed  (2's comp)"  n_bits=CoeffBitWidth  bin_pt=CoeffBitWidth-1  latency=bram_latency  init_zero=on  explicit_period=off  period=1  rst=off  init_reg=0  en=off  dbl_ovrd=off  show_param=on  distributed_mem=on  use_rpm=off  gen_core=off
      settings: xl_area=[0, 0, 0, 0, 0, 0, 0]
  ROM2 : xbsIndex_r3/ROM  depth=2^(PFBSize-n_inputs)  initVector=buf(1*2^(PFBSize-n_inputs) + 1:2*2^(PFBSize-n_inputs))  arith_type="Signed  (2's comp)"  n_bits=CoeffBitWidth  bin_pt=CoeffBitWidth-1  latency=bram_latency  init_zero=on  explicit_period=off  period=1  rst=off  init_reg=0  en=off  dbl_ovrd=off  show_param=on  distributed_mem=on  use_rpm=off  gen_core=off
      settings: xl_area=[0, 0, 0, 0, 0, 0, 0]
  ROM3 : xbsIndex_r3/ROM  depth=2^(PFBSize-n_inputs)  initVector=buf(2*2^(PFBSize-n_inputs) + 1:3*2^(PFBSize-n_inputs))  arith_type="Signed  (2's comp)"  n_bits=CoeffBitWidth  bin_pt=CoeffBitWidth-1  latency=bram_latency  init_zero=on  explicit_period=off  period=1  rst=off  init_reg=0  en=off  dbl_ovrd=off  show_param=on  distributed_mem=on  use_rpm=off  gen_core=off
      settings: xl_area=[0, 0, 0, 0, 0, 0, 0]
  ROM4 : xbsIndex_r3/ROM  depth=2^(PFBSize-n_inputs)  initVector=buf(3*2^(PFBSize-n_inputs) + 1:4*2^(PFBSize-n_inputs))  arith_type="Signed  (2's comp)"  n_bits=CoeffBitWidth  bin_pt=CoeffBitWidth-1  latency=bram_latency  init_zero=on  explicit_period=off  period=1  rst=off  init_reg=0  en=off  dbl_ovrd=off  show_param=on  distributed_mem=on  use_rpm=off  gen_core=off
      settings: xl_area=[0, 0, 0, 0, 0, 0, 0]
  ROM5 : xbsIndex_r3/ROM  depth=2^(PFBSize-n_inputs)  initVector=buf(4*2^(PFBSize-n_inputs) + 1:5*2^(PFBSize-n_inputs))  arith_type="Signed  (2's comp)"  n_bits=CoeffBitWidth  bin_pt=CoeffBitWidth-1  latency=bram_latency  init_zero=on  explicit_period=off  period=1  rst=off  init_reg=0  en=off  dbl_ovrd=off  show_param=on  distributed_mem=on  use_rpm=off  gen_core=off
      settings: xl_area=[0, 0, 0, 0, 0, 0, 0]
  ROM6 : xbsIndex_r3/ROM  depth=2^(PFBSize-n_inputs)  initVector=buf(5*2^(PFBSize-n_inputs) + 1:6*2^(PFBSize-n_inputs))  arith_type="Signed  (2's comp)"  n_bits=CoeffBitWidth  bin_pt=CoeffBitWidth-1  latency=bram_latency  init_zero=on  explicit_period=off  period=1  rst=off  init_reg=0  en=off  dbl_ovrd=off  show_param=on  distributed_mem=on  use_rpm=off  gen_core=off
      settings: xl_area=[0, 0, 0, 0, 0, 0, 0]
  ROM7 : xbsIndex_r3/ROM  depth=2^(PFBSize-n_inputs)  initVector=buf(6*2^(PFBSize-n_inputs) + 1:7*2^(PFBSize-n_inputs))  arith_type="Signed  (2's comp)"  n_bits=CoeffBitWidth  bin_pt=CoeffBitWidth-1  latency=bram_latency  init_zero=on  explicit_period=off  period=1  rst=off  init_reg=0  en=off  dbl_ovrd=off  show_param=on  distributed_mem=on  use_rpm=off  gen_core=off
      settings: xl_area=[0, 0, 0, 0, 0, 0, 0]
  ROM8 : xbsIndex_r3/ROM  depth=2^(PFBSize-n_inputs)  initVector=buf(7*2^(PFBSize-n_inputs) + 1:8*2^(PFBSize-n_inputs))  arith_type="Signed  (2's comp)"  n_bits=CoeffBitWidth  bin_pt=CoeffBitWidth-1  latency=bram_latency  init_zero=on  explicit_period=off  period=1  rst=off  init_reg=0  en=off  dbl_ovrd=off  show_param=on  distributed_mem=on  use_rpm=off  gen_core=off
      settings: xl_area=[0, 0, 0, 0, 0, 0, 0]
  Register : xbsIndex_r3/Register  init=0  reg_only_valid=off  explicit_period=off  period=1  rst=off  en=off  out_en=off  dbl_ovrd=off  show_param=off
      settings: xl_area=[0, 0, 0, 0, 0, 0, 0]
  Reinterpret{1..9} (9 alike) : xbsIndex_r3/Reinterpret  force_arith_type=on  arith_type=Unsigned  force_bin_pt=on  bin_pt=0  force_valid=on
  dout : Outport
  sync_out : Outport  Port=2
  coeff : Outport  Port=3
  wires:
  Reinterpret8/1 -> Concat/8
  ROM8/1 -> Reinterpret8/1
  Reinterpret7/1 -> Concat/7
  ROM7/1 -> Reinterpret7/1
  Reinterpret6/1 -> Concat/6
  ROM6/1 -> Reinterpret6/1
  Reinterpret5/1 -> Concat/5
  ROM5/1 -> Reinterpret5/1
  Reinterpret4/1 -> Concat/4
  ROM4/1 -> Reinterpret4/1
  Reinterpret3/1 -> Concat/3
  ROM3/1 -> Reinterpret3/1
  Reinterpret2/1 -> Concat/2
  ROM2/1 -> Reinterpret2/1
  Reinterpret1/1 -> Concat/1
  ROM1/1 -> Reinterpret1/1
  Counter/1 -> ROM8/1, ROM7/1, ROM6/1, ROM5/1, ROM4/1, ROM3/1, ROM2/1, ROM1/1
  Register/1 -> coeff/1
  Concat/1 -> Register/1
  Delay/1 -> sync_out/1
  sync/1 -> Delay/1, Counter/1
  Delay1/1 -> dout/1
  din/1 -> Reinterpret9/1
  Reinterpret9/1 -> Delay1/1

== system pfb_library/last_tap/c_to_ri ==
  c : Inport  Port=1  LatchInput=off
  Reinterpret : xbsIndex_r3/Reinterpret  force_arith_type=on  arith_type="Signed  (2's comp)"  force_bin_pt=on  bin_pt=BitWidthIn - 1  force_valid=on
  Reinterpret1 : xbsIndex_r3/Reinterpret  force_arith_type=on  arith_type="Signed  (2's comp)"  force_bin_pt=on  bin_pt=BitWidthIn - 1  force_valid=on
  Slice : xbsIndex_r3/Slice  mode=Upper Bit Location + Width  nbits=BitWidthIn  bit1=0  base1=MSB of Input  bit0=0  base0=LSB of Input  boolean_output=off  explicit_period=off  period=1  dbl_ovrd=off
  Slice1 : xbsIndex_r3/Slice  mode=Lower Bit Location + Width  nbits=BitWidthIn  bit1=0  base1=MSB of Input  bit0=0  base0=LSB of Input  boolean_output=off  explicit_period=off  period=1  dbl_ovrd=off
  re : Outport
  im : Outport  Port=2
  wires:
  c/1 -> Slice1/1, Slice/1
  Reinterpret1/1 -> im/1
  Reinterpret/1 -> re/1
  Slice1/1 -> Reinterpret1/1
  Slice/1 -> Reinterpret/1
